simulink model "getAccData"  (R2019b)
settings: Solver=FixedStepAuto  StartTime=0.0  StopTime=10.0  FixedStep=1E-3  RelTol=1e-3
libraries: frdmk64flib x5, nucleoutilitieslib x1
settings Model: ExtModeTrigDuration=5  Creator=scotts24  LastModifiedBy=scotts24
settings DataIOCC: ReturnWorkspaceOutputs=off
settings OptimizationCC: PassReuseOutputArgsThreshold=0  MaxStackSize=64
settings DebuggingCC: ParameterTunabilityLossMsg=error  ArithmeticOperatorsInVariantConditions=warning
settings HardwareCC: ProdBitPerPointer=32  ProdBitPerSizeT=32  ProdBitPerPtrDiffT=32  ProdLargestAtomicInteger=Long  ProdLargestAtomicFloat=Double  ProdWordSize=32  ProdHWDeviceType=ARM Compatible->ARM Cortex  UseEmbeddedCoderFeatures=off
settings SFSimCC: SimUseLocalCustomCode=off  MATLABDynamicMemAlloc=off  CustomCodeUndefinedFunction=UseInterfaceOnly
settings RTWCC: SystemTargetFile=ert.tlc  HardwareBoard=NXP FRDM-K64F  TLCOptions="-aInlineSetEventsForThisBaseRateFcn=TLC_FALSE -aSuppressMultiTaskScheduler=TLC_FALSE  -aRateBasedStepFcn=0"  TemplateMakefile=ert_default_tmf  GenerateReport=on  RTWUseLocalCustomCode=off  Toolchain=GNU Tools for ARM Embedded Processors  LaunchReport=on
settings CodeAppCC: ForceParamTrailComments=on  OperatorAnnotations=on
settings ERTTargetCC: ERTCustomFileBanners=off  SupportContinuousTime=on  SupportNonInlinedSFcns=on  RemoveResetFunc=off  ModelStepFunctionPrototypeControlCompliant=off

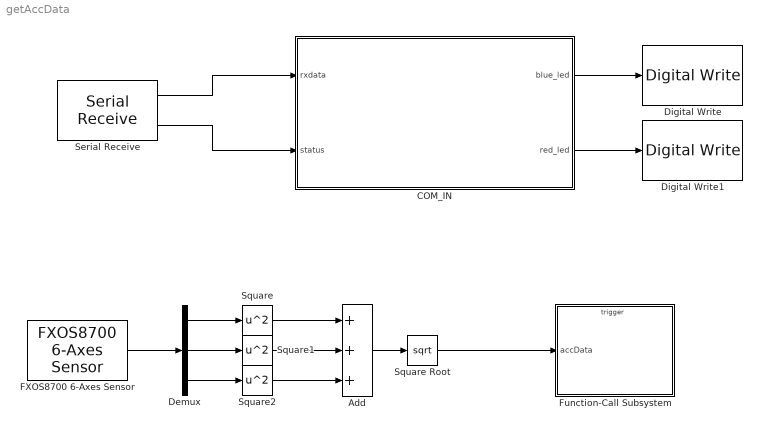
== system getAccData ==
  Add : Sum  Inputs=3  AccumDataTypeStr=double
  COM_IN : Stateflow chart  BlockKeywords=__PRM__SERIALIZED__DATA__:Stateflow Chart,Stateflow Diagram  TreatAsAtomicUnit=on
  Demux : Demux  Outputs=3
  Digital Write : frdmk64flib/Digital Write  Whichpin=BLUE_LED
      settings: SourceProductName=Simulink Coder Support Package for NXP FRDM-K64F Board
  Digital Write1 : frdmk64flib/Digital Write  Whichpin=RED_LED
      settings: SourceProductName=Simulink Coder Support Package for NXP FRDM-K64F Board
  FXOS8700 6-Axes Sensor : frdmk64flib/FXOS8700 6-Axes Sensor  Activesensor=Accelerometer only  ODR=800Hz  HybridODR=400Hz  Accelfullrange=-4g to +4g  SampleTime=-1
      settings: SourceProductName=Simulink Coder Support Package for NXP FRDM-K64F Board
  Function-Call Subsystem : Subsystem  TreatAsAtomicUnit=on
  Serial Receive : frdmk64flib/Serial Receive  SCIModule=0  Baudrate=uint32(9600)  Parity=None  StopBits=1  HardwareFlowControl=None  ByteOrder=LittleEndian  DataType=uint8  DataLength=2  BlockingMode=off  OutputStatus=on  SampleTime=-1
      settings: SourceProductName=Simulink Coder Support Package for NXP FRDM-K64F Board
  Square : Math  Operator=square  SignedPower=off  OutDataTypeStr=double  SaturateOnIntegerOverflow=on
  Square Root : Sqrt  OutDataTypeStr=double  SaturateOnIntegerOverflow=on
  Square1 : Math  Operator=square  SignedPower=off  OutDataTypeStr=double  SaturateOnIntegerOverflow=on
  Square2 : Math  Operator=square  SignedPower=off  OutDataTypeStr=double  SaturateOnIntegerOverflow=on
  wires:
  Serial Receive/1 -> COM_IN/1(rxdata)
  Serial Receive/2 -> COM_IN/2(status)
  FXOS8700 6-Axes Sensor/1 -> Demux/1
  Demux/1 -> Square/1
  Demux/2 -> Square1/1
  Demux/3 -> Square2/1
  Square/1 -> Add/1
  Square1/1 -> Add/2
  Square2/1 -> Add/3
  Add/1 -> Square Root/1
  Square Root/1 -> Function-Call Subsystem/1(accData)
  COM_IN/1(blue_led) -> Digital Write/1
  COM_IN/2(red_led) -> Digital Write1/1

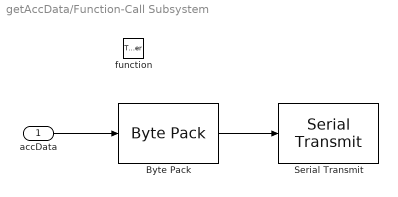
== system getAccData/Function-Call Subsystem ==
  accData : Inport
  function : TriggerPort  TriggerType=function-call  IsSimulinkFunction=on  FunctionName=transmitData  VariantControl=Variant
  Byte Pack : nucleoutilitieslib/Byte Pack  datatypes={'double'}  byteAlign=1  blockPlatform=nucleo
      settings: SourceProductName=Embedded Coder Support Package for ARM Cortex-A Processors  SourceProductBaseCode=ECCORTEXA
  Serial Transmit : frdmk64flib/Serial Transmit  SCIModule=0  Baudrate=uint32(9600)  Parity=None  StopBits=1  HardwareFlowControl=None  ByteOrder=LittleEndian  BlockingMode=on  OutputStatus=off
      settings: SourceProductName=Simulink Coder Support Package for NXP FRDM-K64F Board
  wires:
  accData/1 -> Byte Pack/1
  Byte Pack/1 -> Serial Transmit/1

== stateflow chart getAccData/COM_IN ==
  state TRANSMIT
    entry:
    blue_led = false;
    red_led = true;
    transmitData();
  state INIT
    sampleTime = 100;
    blue_led = true;
    red_led = false;
  TRANSMIT -> TRANSMIT [order 2] : [after(sampleTime,msec)]
  (default) -> INIT
  INIT -> TRANSMIT : [status == 0 && rxdata(1) == hex2dec('16') && rxdata(2) == hex2dec('40')]
  TRANSMIT -> INIT [order 1] : [status == 0 && rxdata(1) == hex2dec('16') && rxdata(2) == hex2dec('45')]
  data: rxdata input uint8; status input uint8; sampleTime local uint16; blue_led output boolean; red_led output boolean
